simulink model "UZ_EnDat_be4_diffrework"  (R2023b)
settings: Solver=FixedStepDiscrete  StartTime=0  StopTime=0.002  RelTol=1e-3
model workspace (MAT data in the model file):
  Select = 0
libraries: hdlsllib x207, simulink x17, simulink_extras x3
(part 2 of 5)

== system UZ_EnDat_be4_diffrework/UZ_ENDAT/CLKCNTER_NOSTOP ==
  CLK : Inport
  CLK2CNT : Inport  Port=2
  ResetCNT : Inport  Port=3  OutDataTypeStr=boolean
  Delay1 : Delay  DelayLength=1
  Positional_Counter : Subsystem  TreatAsAtomicUnit=on
      settings: LibrarySourceBlock=|
      | hdlsllib/Ports &
      | Subsystems/Triggered
      | Subsystem
  SetZero32modified : Subsystem
  CNT : Outport
  wires:
  Delay1/1 -> SetZero32modified/1(valin), CNT/1
  CLK2CNT/1 -> Positional_Counter/Trigger
  ResetCNT/1 -> SetZero32modified/2(setzero)
  Positional_Counter/1(divider) -> Delay1/1
  CLK/1 -> SetZero32modified/Trigger
  SetZero32modified/1(valueout) -> Positional_Counter/1(valueout)

== system UZ_EnDat_be4_diffrework/UZ_ENDAT/CLKCNTER_RAMPUP ==
  CLK : Inport
  CLK2CNT : Inport  Port=2
  ResetCNT : Inport  Port=3  OutDataTypeStr=boolean
  Delay1 : Delay  DelayLength=1
  Positional_Counter : Subsystem  TreatAsAtomicUnit=on
      settings: LibrarySourceBlock=|
      | hdlsllib/Ports &
      | Subsystems/Triggered
      | Subsystem
  SetZero32modified : Subsystem
  CNT : Outport
  wires:
  CLK2CNT/1 -> Positional_Counter/Trigger
  Delay1/1 -> Positional_Counter/1(valueout), CNT/1
  SetZero32modified/1(valueout) -> Delay1/1
  CLK/1 -> SetZero32modified/Trigger
  Positional_Counter/1(divider) -> SetZero32modified/1(valin)
  ResetCNT/1 -> SetZero32modified/2(setzero)

== system UZ_EnDat_be4_diffrework/UZ_ENDAT/CLKDIV1 ==
  CLK1 : Inport  OutDataTypeStr=boolean
  Delay : Delay  DelayLength=1
  Logical Operator1 : Logic  Operator=NOT  AllPortsSameDT=off  OutDataTypeStr=boolean
  Triggered Subsystem : Subsystem  TreatAsAtomicUnit=on
      settings: LibrarySourceBlock=|
      | hdlsllib/Ports &
      | Subsystems/Triggered
      | Subsystem
  CLK/2 : Outport  OutDataTypeStr=boolean  VectorParamsAs1DForOutWhenUnconnected=off
  wires:
  Logical Operator1/1 -> CLK/2/1, Delay/1
  CLK1/1 -> Triggered Subsystem/Trigger
  Triggered Subsystem/1(OUT) -> Logical Operator1/1
  Delay/1 -> Triggered Subsystem/1(IN)

== system UZ_EnDat_be4_diffrework/UZ_ENDAT/CLKDIV2 ==
  CLK1 : Inport  OutDataTypeStr=boolean
  Delay : Delay  DelayLength=1
  Logical Operator1 : Logic  Operator=NOT  AllPortsSameDT=off  OutDataTypeStr=boolean
  Triggered Subsystem : Subsystem  TreatAsAtomicUnit=on
      settings: LibrarySourceBlock=|
      | hdlsllib/Ports &
      | Subsystems/Triggered
      | Subsystem
  CLK/2 : Outport  OutDataTypeStr=boolean  VectorParamsAs1DForOutWhenUnconnected=off
  wires:
  Logical Operator1/1 -> CLK/2/1, Delay/1
  CLK1/1 -> Triggered Subsystem/Trigger
  Triggered Subsystem/1(OUT) -> Logical Operator1/1
  Delay/1 -> Triggered Subsystem/1(IN)

== system UZ_EnDat_be4_diffrework/UZ_ENDAT/CLKDIV3 ==
  CLK1 : Inport  OutDataTypeStr=boolean
  Delay : Delay  DelayLength=1
  Logical Operator1 : Logic  Operator=NOT  AllPortsSameDT=off  OutDataTypeStr=boolean
  Triggered Subsystem : Subsystem  TreatAsAtomicUnit=on
      settings: LibrarySourceBlock=|
      | hdlsllib/Ports &
      | Subsystems/Triggered
      | Subsystem
  CLK/2 : Outport  OutDataTypeStr=boolean  VectorParamsAs1DForOutWhenUnconnected=off
  wires:
  Logical Operator1/1 -> CLK/2/1, Delay/1
  CLK1/1 -> Triggered Subsystem/Trigger
  Triggered Subsystem/1(OUT) -> Logical Operator1/1
  Delay/1 -> Triggered Subsystem/1(IN)

== system UZ_EnDat_be4_diffrework/UZ_ENDAT/CLKDIV4 ==
  CLK1 : Inport  OutDataTypeStr=boolean
  Delay : Delay  DelayLength=1
  Logical Operator1 : Logic  Operator=NOT  AllPortsSameDT=off  OutDataTypeStr=boolean
  Triggered Subsystem : Subsystem  TreatAsAtomicUnit=on
      settings: LibrarySourceBlock=|
      | hdlsllib/Ports &
      | Subsystems/Triggered
      | Subsystem
  CLK/2 : Outport  OutDataTypeStr=boolean  VectorParamsAs1DForOutWhenUnconnected=off
  wires:
  Logical Operator1/1 -> CLK/2/1, Delay/1
  CLK1/1 -> Triggered Subsystem/Trigger
  Triggered Subsystem/1(OUT) -> Logical Operator1/1
  Delay/1 -> Triggered Subsystem/1(IN)

== system UZ_EnDat_be4_diffrework/UZ_ENDAT/CLKDIV5 ==
  CLK1 : Inport  OutDataTypeStr=boolean
  Delay : Delay  DelayLength=1
  Logical Operator1 : Logic  Operator=NOT  AllPortsSameDT=off  OutDataTypeStr=boolean
  Triggered Subsystem : Subsystem  TreatAsAtomicUnit=on
      settings: LibrarySourceBlock=|
      | hdlsllib/Ports &
      | Subsystems/Triggered
      | Subsystem
  CLK/2 : Outport  OutDataTypeStr=boolean  VectorParamsAs1DForOutWhenUnconnected=off
  wires:
  Logical Operator1/1 -> CLK/2/1, Delay/1
  CLK1/1 -> Triggered Subsystem/Trigger
  Triggered Subsystem/1(OUT) -> Logical Operator1/1
  Delay/1 -> Triggered Subsystem/1(IN)

== system UZ_EnDat_be4_diffrework/UZ_ENDAT/CLKDIV6 ==
  CLK1 : Inport  OutDataTypeStr=boolean
  Delay : Delay  DelayLength=1
  Logical Operator1 : Logic  Operator=NOT  AllPortsSameDT=off  OutDataTypeStr=boolean
  Triggered Subsystem : Subsystem  TreatAsAtomicUnit=on
      settings: LibrarySourceBlock=|
      | hdlsllib/Ports &
      | Subsystems/Triggered
      | Subsystem
  CLK/2 : Outport  OutDataTypeStr=boolean  VectorParamsAs1DForOutWhenUnconnected=off
  wires:
  Logical Operator1/1 -> CLK/2/1, Delay/1
  CLK1/1 -> Triggered Subsystem/Trigger
  Triggered Subsystem/1(OUT) -> Logical Operator1/1
  Delay/1 -> Triggered Subsystem/1(IN)

== system UZ_EnDat_be4_diffrework/UZ_ENDAT/CLKDIV7 ==
  CLK1 : Inport  OutDataTypeStr=boolean
  Delay : Delay  DelayLength=1
  Logical Operator1 : Logic  Operator=NOT  AllPortsSameDT=off  OutDataTypeStr=boolean
  Triggered Subsystem : Subsystem  TreatAsAtomicUnit=on
      settings: LibrarySourceBlock=|
      | hdlsllib/Ports &
      | Subsystems/Triggered
      | Subsystem
  CLK/2 : Outport  OutDataTypeStr=boolean  VectorParamsAs1DForOutWhenUnconnected=off
  wires:
  Logical Operator1/1 -> CLK/2/1, Delay/1
  CLK1/1 -> Triggered Subsystem/Trigger
  Triggered Subsystem/1(OUT) -> Logical Operator1/1
  Delay/1 -> Triggered Subsystem/1(IN)

== system UZ_EnDat_be4_diffrework/UZ_ENDAT/CLKDIV8 ==
  CLK1 : Inport  OutDataTypeStr=boolean
  Delay : Delay  DelayLength=1
  Logical Operator1 : Logic  Operator=NOT  AllPortsSameDT=off  OutDataTypeStr=boolean
  Triggered Subsystem : Subsystem  TreatAsAtomicUnit=on
      settings: LibrarySourceBlock=|
      | hdlsllib/Ports &
      | Subsystems/Triggered
      | Subsystem
  CLK/2 : Outport  OutDataTypeStr=boolean  VectorParamsAs1DForOutWhenUnconnected=off
  wires:
  Logical Operator1/1 -> CLK/2/1, Delay/1
  CLK1/1 -> Triggered Subsystem/Trigger
  Triggered Subsystem/1(OUT) -> Logical Operator1/1
  Delay/1 -> Triggered Subsystem/1(IN)

== system UZ_EnDat_be4_diffrework/UZ_ENDAT/CLKDIV9 ==
  CLK1 : Inport  OutDataTypeStr=boolean
  Delay : Delay  DelayLength=1
  Logical Operator1 : Logic  Operator=NOT  AllPortsSameDT=off  OutDataTypeStr=boolean
  Triggered Subsystem : Subsystem  TreatAsAtomicUnit=on
      settings: LibrarySourceBlock=|
      | hdlsllib/Ports &
      | Subsystems/Triggered
      | Subsystem
  CLK/2 : Outport  OutDataTypeStr=boolean  VectorParamsAs1DForOutWhenUnconnected=off
  wires:
  Logical Operator1/1 -> CLK/2/1, Delay/1
  CLK1/1 -> Triggered Subsystem/Trigger
  Triggered Subsystem/1(OUT) -> Logical Operator1/1
  Delay/1 -> Triggered Subsystem/1(IN)

== system UZ_EnDat_be4_diffrework/UZ_ENDAT/CONTROLWORDRAW ==
  CLK : Inport
  DATA : Inport  Port=2
  WORDTOBOOL : Subsystem  TreatAsAtomicUnit=on
  DATAOUT0 : Outport  VectorParamsAs1DForOutWhenUnconnected=off
  DATAOUT1 : Outport  Port=2  VectorParamsAs1DForOutWhenUnconnected=off
  DATAOUT2 : Outport  Port=3  VectorParamsAs1DForOutWhenUnconnected=off
  DATAOUT3 : Outport  Port=4  VectorParamsAs1DForOutWhenUnconnected=off
  DATAOUT4 : Outport  Port=5  VectorParamsAs1DForOutWhenUnconnected=off
  DATAOUT5 : Outport  Port=6  VectorParamsAs1DForOutWhenUnconnected=off
  DATAOUT6 : Outport  Port=7  VectorParamsAs1DForOutWhenUnconnected=off
  DATAOUT7 : Outport  Port=8  VectorParamsAs1DForOutWhenUnconnected=off
  DATAOUT8 : Outport  Port=9  VectorParamsAs1DForOutWhenUnconnected=off
  DATAOUT9 : Outport  Port=10  VectorParamsAs1DForOutWhenUnconnected=off
  DATAOUT10 : Outport  Port=11  VectorParamsAs1DForOutWhenUnconnected=off
  DATAOUT11 : Outport  Port=12  VectorParamsAs1DForOutWhenUnconnected=off
  DATAOUT12 : Outport  Port=13  VectorParamsAs1DForOutWhenUnconnected=off
  DATAOUT13 : Outport  Port=14  VectorParamsAs1DForOutWhenUnconnected=off
  DATAOUT14 : Outport  Port=15  VectorParamsAs1DForOutWhenUnconnected=off
  DATAOUT15 : Outport  Port=16  VectorParamsAs1DForOutWhenUnconnected=off
  wires:
  DATA/1 -> WORDTOBOOL/1(DATAIN)
  CLK/1 -> WORDTOBOOL/Trigger
  WORDTOBOOL/1(DATAOUT0) -> DATAOUT0/1
  WORDTOBOOL/2(DATAOUT1) -> DATAOUT1/1
  WORDTOBOOL/3(DATAOUT2) -> DATAOUT2/1
  WORDTOBOOL/4(DATAOUT3) -> DATAOUT3/1
  WORDTOBOOL/6(DATAOUT5) -> DATAOUT5/1
  WORDTOBOOL/5(DATAOUT4) -> DATAOUT4/1
  WORDTOBOOL/7(DATAOUT6) -> DATAOUT6/1
  WORDTOBOOL/8(DATAOUT7) -> DATAOUT7/1
  WORDTOBOOL/10(DATAOUT9) -> DATAOUT9/1
  WORDTOBOOL/9(DATAOUT8) -> DATAOUT8/1
  WORDTOBOOL/11(DATAOUT10) -> DATAOUT10/1
  WORDTOBOOL/12(DATAOUT11) -> DATAOUT11/1
  WORDTOBOOL/14(DATAOUT13) -> DATAOUT13/1
  WORDTOBOOL/13(DATAOUT12) -> DATAOUT12/1
  WORDTOBOOL/15(DATAOUT14) -> DATAOUT14/1
  WORDTOBOOL/16(DATAOUT15) -> DATAOUT15/1

== system UZ_EnDat_be4_diffrework/UZ_ENDAT/CONTROLWORDSTORED ==
  CLK : Inport
  DATA : Inport  Port=2
  WORDTOBOOL : Subsystem  TreatAsAtomicUnit=on
  DATAOUT0 : Outport  VectorParamsAs1DForOutWhenUnconnected=off
  DATAOUT1 : Outport  Port=2  VectorParamsAs1DForOutWhenUnconnected=off
  DATAOUT2 : Outport  Port=3  VectorParamsAs1DForOutWhenUnconnected=off
  DATAOUT3 : Outport  Port=4  VectorParamsAs1DForOutWhenUnconnected=off
  DATAOUT4 : Outport  Port=5  VectorParamsAs1DForOutWhenUnconnected=off
  DATAOUT5 : Outport  Port=6  VectorParamsAs1DForOutWhenUnconnected=off
  DATAOUT6 : Outport  Port=7  VectorParamsAs1DForOutWhenUnconnected=off
  DATAOUT7 : Outport  Port=8  VectorParamsAs1DForOutWhenUnconnected=off
  DATAOUT8 : Outport  Port=9  VectorParamsAs1DForOutWhenUnconnected=off
  DATAOUT9 : Outport  Port=10  VectorParamsAs1DForOutWhenUnconnected=off
  DATAOUT10 : Outport  Port=11  VectorParamsAs1DForOutWhenUnconnected=off
  DATAOUT11 : Outport  Port=12  VectorParamsAs1DForOutWhenUnconnected=off
  DATAOUT12 : Outport  Port=13  VectorParamsAs1DForOutWhenUnconnected=off
  DATAOUT13 : Outport  Port=14  VectorParamsAs1DForOutWhenUnconnected=off
  DATAOUT14 : Outport  Port=15  VectorParamsAs1DForOutWhenUnconnected=off
  DATAOUT15 : Outport  Port=16  VectorParamsAs1DForOutWhenUnconnected=off
  wires:
  DATA/1 -> WORDTOBOOL/1(DATAIN)
  CLK/1 -> WORDTOBOOL/Trigger
  WORDTOBOOL/1(DATAOUT0) -> DATAOUT0/1
  WORDTOBOOL/2(DATAOUT1) -> DATAOUT1/1
  WORDTOBOOL/3(DATAOUT2) -> DATAOUT2/1
  WORDTOBOOL/4(DATAOUT3) -> DATAOUT3/1
  WORDTOBOOL/6(DATAOUT5) -> DATAOUT5/1
  WORDTOBOOL/5(DATAOUT4) -> DATAOUT4/1
  WORDTOBOOL/7(DATAOUT6) -> DATAOUT6/1
  WORDTOBOOL/8(DATAOUT7) -> DATAOUT7/1
  WORDTOBOOL/10(DATAOUT9) -> DATAOUT9/1
  WORDTOBOOL/9(DATAOUT8) -> DATAOUT8/1
  WORDTOBOOL/11(DATAOUT10) -> DATAOUT10/1
  WORDTOBOOL/12(DATAOUT11) -> DATAOUT11/1
  WORDTOBOOL/14(DATAOUT13) -> DATAOUT13/1
  WORDTOBOOL/13(DATAOUT12) -> DATAOUT12/1
  WORDTOBOOL/15(DATAOUT14) -> DATAOUT14/1
  WORDTOBOOL/16(DATAOUT15) -> DATAOUT15/1

== system UZ_EnDat_be4_diffrework/UZ_ENDAT/CRC_Check ==
  set : Inport
  data : Inport  Port=2  OutDataTypeStr=boolean
  clk : Inport  Port=3  OutDataTypeStr=boolean
  Constant : Constant  OutDataTypeStr=boolean  SampleTime=-1
  Constant1 : Constant  Value=0  OutDataTypeStr=boolean  SampleTime=-1
  DFF1 : Subsystem
  DFF2 : Subsystem
  DFF3 : Subsystem
  DFF4 : Subsystem
  DFF5 : Subsystem
  DFF6 : Subsystem  Commented=on
  FF0 : Subsystem  Commented=on  TreatAsAtomicUnit=on
      settings: LibrarySourceBlock=|
      | hdlsllib/Ports &
      | Subsystems/Triggered
      | Subsystem
  Logical Operator : Logic  Operator=OR  AllPortsSameDT=off  OutDataTypeStr=boolean
  Logical Operator{1..2,5..6} (4 alike) : Logic  AllPortsSameDT=off  OutDataTypeStr=boolean
  Logical Operator3 : Logic  Operator=NOT  AllPortsSameDT=off  OutDataTypeStr=boolean
  Logical Operator4 : Logic  Operator=NOT  AllPortsSameDT=off  OutDataTypeStr=boolean
  Memory : Memory  InheritSampleTime=on
  Memory1 : Memory  InheritSampleTime=on
  Relational Operator : RelationalOperator  Operator===  OutDataTypeStr=boolean  InputSameDT=off
  Relational Operator1 : RelationalOperator  Operator===  OutDataTypeStr=boolean  InputSameDT=off
  Relational Operator2 : RelationalOperator  Operator===  OutDataTypeStr=boolean  InputSameDT=off
  Terminator{,1..3} (4 alike) : Terminator
  crc : Outport
  CRC1 : Outport  Port=2
  CRC2 : Outport  Port=3
  CRC3 : Outport  Port=4
  CRC4 : Outport  Port=5
  CRC5 : Outport  Port=6
  wires:
  Logical Operator/1 -> crc/1
  Logical Operator2/1 -> Logical Operator/2
  Logical Operator1/1 -> Logical Operator/1
  data/1 -> Relational Operator/2, Logical Operator1/1
  Logical Operator3/1 -> Logical Operator1/2
  Logical Operator4/1 -> Logical Operator3/1, Logical Operator2/2
  Logical Operator5/1 -> Memory1/1
  Relational Operator/1 -> DFF1/3(D), Logical Operator6/1
  clk/1 -> DFF1/2(CLK), DFF2/2(CLK), DFF3/2(CLK), DFF5/2(CLK), DFF4/2(CLK)
  set/1 -> Logical Operator6/2, Logical Operator5/2, Logical Operator4/1
  DFF1/1(OQ) -> Relational Operator1/1, CRC1/1
  Logical Operator6/1 -> Memory/1
  Relational Operator1/1 -> DFF2/3(D)
  Relational Operator2/1 -> DFF4/3(D)
  DFF3/1(OQ) -> CRC3/1, Relational Operator2/1
  DFF4/1(OQ) -> DFF5/3(D), CRC4/1
  DFF5/2(NOQ) -> Logical Operator2/1
  DFF5/1(OQ) -> Logical Operator5/1, CRC5/1
  DFF2/1(OQ) -> DFF3/3(D), CRC2/1
  DFF1/2(NOQ) -> Terminator/1
  DFF2/2(NOQ) -> Terminator1/1
  DFF3/2(NOQ) -> Terminator2/1
  DFF4/2(NOQ) -> Terminator3/1
  Constant/1 -> DFF3/1(SET), DFF5/1(SET), DFF4/1(SET), DFF2/1(SET), DFF1/1(SET)
  Constant1/1 -> DFF5/4(RST), DFF4/4(RST), DFF3/4(RST), DFF2/4(RST), DFF1/4(RST)
  Memory/1 -> Relational Operator2/2, Relational Operator1/2
  Memory1/1 -> Relational Operator/1

== system UZ_EnDat_be4_diffrework/UZ_ENDAT/DATA2CLOCKSYNCER ==
  In1 : Inport
  FAKTOR : Inport  Port=2
  Constant : Constant  Value=100  OutDataTypeStr=uint16  SampleTime=-1
  Constant1 : Constant  Value=45  OutDataTypeStr=uint16  SampleTime=-1
  Constant2 : Constant  Value=2  OutDataTypeStr=uint16  SampleTime=-1
  Constant23 : Constant  Value=20  OutDataTypeStr=uint16  SampleTime=-1
  Constant24 : Constant  Value=29  OutDataTypeStr=uint16  SampleTime=-1
  Constant3 : Constant  Value=12  OutDataTypeStr=uint16  SampleTime=-1
  Constant4 : Constant  Value=4  OutDataTypeStr=uint16  SampleTime=-1
  Constant7 : Constant  Value=8  OutDataTypeStr=uint16  SampleTime=-1
  Display15 : Display
  Divide : Product  Inputs=*/  OutDataTypeStr=uint16  RndMeth=Simplest  SaturateOnIntegerOverflow=on  LockScale=on
  Multiport Switch1 : MultiPortSwitch  DataPortOrder=Zero-based contiguous  Inputs=7  DataPortIndices={8,16,32,64}  zeroidx=on  SaturateOnIntegerOverflow=off  InputSameDT=off
  Product : Product  RndMeth=Simplest  SaturateOnIntegerOverflow=on  OutDataTypeStr=Inherit: Same as first input
  Out1 : Outport
  wires:
  In1/1 -> Multiport Switch1/1
  FAKTOR/1 -> Product/2
  Constant/1 -> Divide/2
  Multiport Switch1/1 -> Product/1
  Product/1 -> Divide/1
  Constant2/1 -> Multiport Switch1/2
  Constant4/1 -> Multiport Switch1/3
  Constant7/1 -> Multiport Switch1/4
  Constant3/1 -> Multiport Switch1/5
  Constant23/1 -> Multiport Switch1/6
  Constant24/1 -> Multiport Switch1/7
  Constant1/1 -> Multiport Switch1/8
  Divide/1 -> Display15/1, Out1/1

== system UZ_EnDat_be4_diffrework/UZ_ENDAT/DATA2CLOCKSYNCER1 ==
  In1 : Inport
  FAKTOR : Inport  Port=2
  Constant : Constant  Value=9999  OutDataTypeStr=uint16  SampleTime=-1
  Constant1 : Constant  Value=384  OutDataTypeStr=uint16  SampleTime=-1
  Constant2 : Constant  Value=5  OutDataTypeStr=uint16  SampleTime=-1
  Constant23 : Constant  Value=96  OutDataTypeStr=uint16  SampleTime=-1
  Constant24 : Constant  Value=192  OutDataTypeStr=uint16  SampleTime=-1
  Constant3 : Constant  Value=48  OutDataTypeStr=uint16  SampleTime=-1
  Constant4 : Constant  Value=11  OutDataTypeStr=uint16  SampleTime=-1
  Constant7 : Constant  Value=23  OutDataTypeStr=uint16  SampleTime=-1
  Display15 : Display
  Divide : Product  Inputs=*/  OutDataTypeStr=uint16  RndMeth=Simplest  SaturateOnIntegerOverflow=on  LockScale=on
  Multiport Switch1 : MultiPortSwitch  DataPortOrder=Zero-based contiguous  Inputs=7  DataPortIndices={8,16,32,64}  zeroidx=on  SaturateOnIntegerOverflow=off  InputSameDT=off
  Product : Product  RndMeth=Simplest  SaturateOnIntegerOverflow=on  OutDataTypeStr=Inherit: Same as first input
  Out1 : Outport
  wires:
  In1/1 -> Multiport Switch1/1
  FAKTOR/1 -> Product/2
  Constant/1 -> Divide/2
  Multiport Switch1/1 -> Product/1
  Product/1 -> Divide/1
  Constant2/1 -> Multiport Switch1/2
  Constant4/1 -> Multiport Switch1/3
  Constant7/1 -> Multiport Switch1/4
  Constant3/1 -> Multiport Switch1/5
  Constant23/1 -> Multiport Switch1/6
  Constant24/1 -> Multiport Switch1/7
  Constant1/1 -> Multiport Switch1/8
  Divide/1 -> Display15/1, Out1/1

== system UZ_EnDat_be4_diffrework/UZ_ENDAT/DATAFLOWCHGER ==
  CLKSEL : Inport
  FACTOR : Inport  Port=2
  Constant : Constant  Value=100  OutDataTypeStr=uint16  SampleTime=-1
  Constant{14..18,27..28} (7 alike) : Constant  Value=10  OutDataTypeStr=uint16  SampleTime=-1
  Divide : Product  Inputs=*/  InputSameDT=on  OutDataTypeStr=uint16  RndMeth=Simplest  SaturateOnIntegerOverflow=on
  Multiport Switch2 : MultiPortSwitch  DataPortOrder=Zero-based contiguous  Inputs=7  DataPortIndices={8,16,32,64}  zeroidx=on  SaturateOnIntegerOverflow=off  InputSameDT=off
  Product : Product  RndMeth=Simplest  SaturateOnIntegerOverflow=on  OutDataTypeStr=Inherit: Same as first input
  Output : Outport
  wires:
  Product/1 -> Divide/1
  CLKSEL/1 -> Multiport Switch2/1
  FACTOR/1 -> Product/2
  Constant/1 -> Divide/2
  Divide/1 -> Output/1
  Multiport Switch2/1 -> Product/1
  Constant15/1 -> Multiport Switch2/2
  Constant16/1 -> Multiport Switch2/3
  Constant17/1 -> Multiport Switch2/4
  Constant18/1 -> Multiport Switch2/5
  Constant27/1 -> Multiport Switch2/6
  Constant28/1 -> Multiport Switch2/7
  Constant14/1 -> Multiport Switch2/8

== system UZ_EnDat_be4_diffrework/UZ_ENDAT/INITIALOFF ==
  CLKAUX : Inport
  CLK : Inport  Port=2
  DATAWR : Inport  Port=3
  DATA : Inport  Port=4
  CLKWR : Inport  Port=5
  FACTOR : Inport  Port=6
  CLKCNTER_FAST : Subsystem
      settings: LibrarySourceBlock=|
      | hdlsllib/Ports &
      | Subsystems/Subsystem
  Constant : Constant  Value=0  OutDataTypeStr=boolean  SampleTime=-1
  Multiport Switch{,1..3} (4 alike) : MultiPortSwitch  DataPortOrder=Zero-based contiguous  Inputs=2  zeroidx=on  SaturateOnIntegerOverflow=off  InputSameDT=off
  Relational Operator : RelationalOperator  Operator=<  OutDataTypeStr=boolean  InputSameDT=off
  Subsystem6 : Subsystem
  CLK_OUT : Outport
  DATAWR_OUT : Outport  Port=2
  DATA_OUT : Outport  Port=3
  CLKWR_OUT : Outport  Port=4
  wires:
  CLKCNTER_FAST/1(CNT) -> Relational Operator/1
  Relational Operator/1 -> Multiport Switch3/1, Multiport Switch2/1, Multiport Switch1/1, Multiport Switch/1
  CLK/1 -> Multiport Switch/2
  Multiport Switch/1 -> CLK_OUT/1
  CLKAUX/1 -> CLKCNTER_FAST/1(CLK)
  Constant/1 -> Multiport Switch3/3, Multiport Switch2/3, Multiport Switch1/3, Multiport Switch/3
  Multiport Switch1/1 -> DATAWR_OUT/1
  Multiport Switch2/1 -> DATA_OUT/1
  Multiport Switch3/1 -> CLKWR_OUT/1
  DATAWR/1 -> Multiport Switch1/2
  DATA/1 -> Multiport Switch2/2
  CLKWR/1 -> Multiport Switch3/2
  Subsystem6/1(out) -> Relational Operator/2
  FACTOR/1 -> Subsystem6/1(FACTOR)

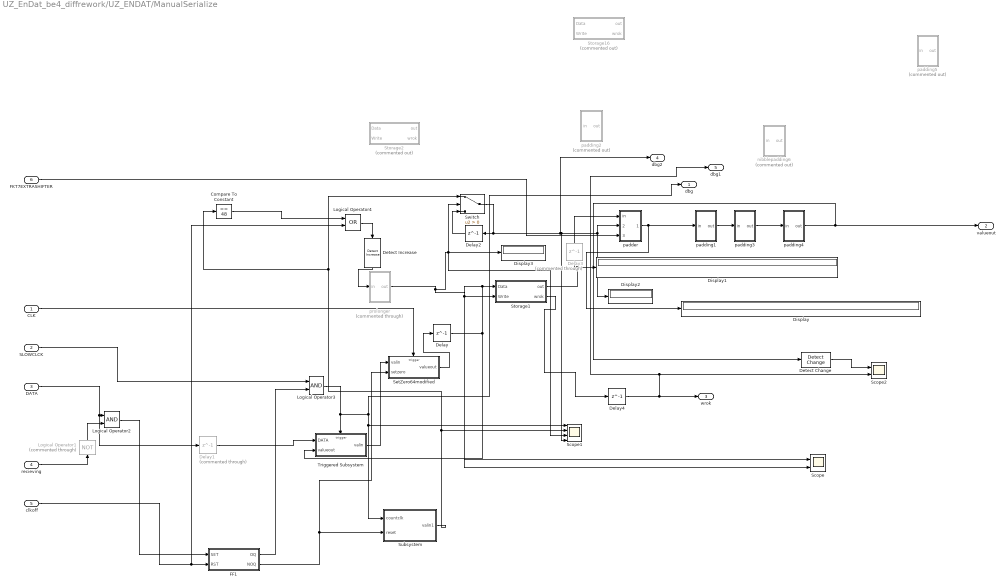
== system UZ_EnDat_be4_diffrework/UZ_ENDAT/ManualSerialize ==
  CLK : Inport
  SLOWCLCK : Inport  Port=2
  DATA : Inport  Port=3
  recieving : Inport  Port=4  OutMin=0  OutMax=1  OutDataTypeStr=boolean
  clkoff : Inport  Port=5  OutMin=0  OutMax=1  OutDataTypeStr=boolean
  FKT7EXTRASHIFTER : Inport  Port=6
  Compare To Constant : hdlsllib/Logic and Bit Operations/Compare To Constant  relop===  const=48  OutDataTypeStr=boolean
  Delay : Delay  DelayLength=1
  Delay1 : Delay  Commented=through  DelayLength=1
  Delay2 : Delay  DelayLength=1
  Delay3 : Delay  Commented=through  DelayLength=1
  Delay4 : Delay  DelayLength=1
  Detect Change : simulink/Logic and Bit Operations/Detect Change  vinit=0  OutDataTypeStr=boolean
  Detect Increase : simulink/Logic and Bit Operations/Detect Increase  vinit=0.0  OutDataTypeStr=boolean
      settings: LibrarySourceBlock=|
      | hdlsllib/Logic and Bit
      | Operations/Detect
      | Increase
  Display{,1..3} (4 alike) : Display
      Display settings: Format=binary (Stored Integer)
      Display1 settings: Format=binary (Stored Integer)
  FF1 : Subsystem  TreatAsAtomicUnit=on
      settings: LibrarySourceBlock=|
      | hdlsllib/Ports &
      | Subsystems/Triggered
      | Subsystem
  Logical Operator1 : Logic  Commented=through  Operator=NOT  AllPortsSameDT=off  OutDataTypeStr=boolean
  Logical Operator2 : Logic  AllPortsSameDT=off  OutDataTypeStr=boolean
  Logical Operator3 : Logic  AllPortsSameDT=off  OutDataTypeStr=boolean
  Logical Operator4 : Logic  Operator=OR  AllPortsSameDT=off  OutDataTypeStr=boolean
  Scope : Scope  NumInputPorts=2
  Scope1 : Scope  NumInputPorts=4
  Scope2 : Scope  NumInputPorts=2
  SetZero64modified : Subsystem
  Storage1 : Subsystem
      settings: LibrarySourceBlock=|
      | hdlsllib/Ports &
      | Subsystems/Subsystem
  Storage16 : Subsystem  Commented=on
      settings: LibrarySourceBlock=|
      | hdlsllib/Ports &
      | Subsystems/Subsystem
  Storage2 : Subsystem  Commented=on
      settings: LibrarySourceBlock=|
      | hdlsllib/Ports &
      | Subsystems/Subsystem
  Subsystem : Subsystem
  Switch : Switch  Criteria=u2 > Threshold  SaturateOnIntegerOverflow=off  InputSameDT=off
  Triggered Subsystem : Subsystem  TreatAsAtomicUnit=on
      settings: LibrarySourceBlock=|
      | hdlsllib/Ports &
      | Subsystems/Triggered
      | Subsystem
  nibblepadding6 : Subsystem  Commented=on
  padder : Subsystem
  padding1 : Subsystem
  padding2 : Subsystem  Commented=on
  padding3 : Subsystem
  padding4 : Subsystem
  padding5 : Subsystem  Commented=on
  prolonger : Subsystem  Commented=through
  dbg : Outport  OutDataTypeStr=boolean  VectorParamsAs1DForOutWhenUnconnected=off
  valueout : Outport  Port=2  OutDataTypeStr=uint64
  wrok : Outport  Port=3  OutDataTypeStr=boolean
  dbg2 : Outport  Port=4  OutDataTypeStr=uint8  VectorParamsAs1DForOutWhenUnconnected=off
  dbg1 : Outport  Port=5  OutDataTypeStr=boolean  VectorParamsAs1DForOutWhenUnconnected=off
  wires:
  SetZero64modified/1(valueout) -> Delay/1
  CLK/1 -> SetZero64modified/Trigger
  SLOWCLCK/1 -> Logical Operator3/1
  Triggered Subsystem/1(valin) -> SetZero64modified/1(valin)
  Storage1/2(wrok) -> Delay4/1
  Logical Operator3/1 -> dbg/1, Subsystem/1(countclk), Scope1/1, Triggered Subsystem/Trigger
  Logical Operator2/1 -> FF1/1(SET)
  FF1/1(OQ) -> Logical Operator3/2
  Logical Operator1/1 -> Logical Operator2/2
  recieving/1 -> Logical Operator1/1
  FF1/2(NOQ) -> Subsystem/2(reset), SetZero64modified/2(setzero)
  DATA/1 -> Delay1/1, Logical Operator2/1
  Compare To Constant/1 -> Logical Operator4/1
  Delay2/1 -> Switch/3
  clkoff/1 -> Logical Operator4/2, FF1/2(RST)
  Logical Operator4/1 -> Detect Increase/1
  Subsystem/1(valin1) -> Scope1/2, Switch/1, Compare To Constant/1
  Delay1/1 -> Triggered Subsystem/1(DATA)
  Delay/1 -> Storage1/1(Data), Scope/2, Triggered Subsystem/2(valueout)
  padding1/1(out) -> padding3/1(in)
  padder/1(out) -> padding1/1(in), Display/1
  Storage1/1(out) -> Delay3/1, Display1/1
  padding3/1(out) -> padding4/1(in)
  Delay3/1 -> padder/1(in)
  prolonger/1(out) -> Storage1/2(Write), Scope/1, Switch/2, Scope1/3, Display3/1
  Detect Increase/1 -> prolonger/1(in)
  padding4/1(out) -> Detect Change/1, valueout/1
  Switch/1 -> Delay2/1, Scope1/4, padder/2(CTR), Display2/1, dbg2/1
  Detect Change/1 -> Scope2/1
  Delay4/1 -> dbg1/1, Scope2/2, wrok/1
  FKT7EXTRASHIFTER/1 -> padder/3(in1)

== system UZ_EnDat_be4_diffrework/UZ_ENDAT/OUTPUTCONTROLCONTINIOUS ==
  CLKCNT : Inport
  CLKS2DATAFLOWCHG : Inport  Port=2
  CLK2ENDOFTRANSMISSION : Inport  Port=3
  OPENCOM : Inport  Port=4
  CLKCNTNOSTOP : Inport  Port=5
  RECOVERYTIME : Inport  Port=6  OutDataTypeStr=uint16
  Add : Sum  OutDataTypeStr=uint16  AccumDataTypeStr=uint16
  Constant : Constant  Value=0  OutDataTypeStr=uint8  SampleTime=-1
  Logical Operator : Logic  Operator=OR  AllPortsSameDT=off  OutDataTypeStr=boolean
  Logical Operator1 : Logic  AllPortsSameDT=off  OutDataTypeStr=boolean
  Logical Operator6 : Logic  Operator=NOT  Inputs=3  AllPortsSameDT=off  OutDataTypeStr=boolean
  Relational Operator : RelationalOperator  Operator=<=  OutDataTypeStr=boolean  InputSameDT=off
  Relational Operator1 : RelationalOperator  OutDataTypeStr=boolean  InputSameDT=off
  Relational Operator2 : RelationalOperator  OutDataTypeStr=boolean  InputSameDT=off
  Relational Operator3 : RelationalOperator  OutDataTypeStr=boolean  InputSameDT=off
  CLKOFF : Outport  OutDataTypeStr=boolean
  DATAINV : Outport  Port=2  OutDataTypeStr=boolean
  RESETCNT : Outport  Port=3  OutDataTypeStr=boolean
  wires:
  CLKCNT/1 -> Relational Operator1/1, Relational Operator2/1, Relational Operator/1
  CLKS2DATAFLOWCHG/1 -> Relational Operator/2
  Relational Operator/1 -> Logical Operator1/1
  CLK2ENDOFTRANSMISSION/1 -> Add/1, Relational Operator1/2
  Relational Operator1/1 -> Logical Operator/2
  Logical Operator/1 -> CLKOFF/1
  OPENCOM/1 -> Logical Operator6/1
  Logical Operator6/1 -> Logical Operator/1
  Relational Operator2/1 -> Logical Operator1/2
  Constant/1 -> Relational Operator2/2
  Logical Operator1/1 -> DATAINV/1
  RECOVERYTIME/1 -> Add/2
  Add/1 -> Relational Operator3/2
  Relational Operator3/1 -> RESETCNT/1
  CLKCNTNOSTOP/1 -> Relational Operator3/1

== system UZ_EnDat_be4_diffrework/UZ_ENDAT/RECOVERYTIMESELECTOR ==
  note: 200khz = 6
      | 1,5mhz = 12
      | 3 mhz = 8
  In1 : Inport
  FAKTOR : Inport  Port=2
  Constant : Constant  Value=100  OutDataTypeStr=uint16  SampleTime=-1
  Constant19 : Constant  Value=96  OutDataTypeStr=uint16  SampleTime=-1
  Constant20 : Constant  Value=48  OutDataTypeStr=uint16  SampleTime=-1
  Constant21 : Constant  Value=192  OutDataTypeStr=uint16  SampleTime=-1
  Constant22 : Constant  Value=255  OutDataTypeStr=uint16  SampleTime=-1
  Constant25 : Constant  Value=24  OutDataTypeStr=uint16  SampleTime=-1
  Constant26 : Constant  Value=12  OutDataTypeStr=uint16  SampleTime=-1
  Constant5 : Constant  Value=6  OutDataTypeStr=uint16  SampleTime=-1
  Divide : Product  Inputs=*/  InputSameDT=on  OutDataTypeStr=uint16  RndMeth=Simplest  SaturateOnIntegerOverflow=on
  Multiport Switch3 : MultiPortSwitch  DataPortOrder=Zero-based contiguous  Inputs=7  DataPortIndices={8,16,32,64}  zeroidx=on  SaturateOnIntegerOverflow=off  InputSameDT=off
  Product : Product  RndMeth=Simplest  SaturateOnIntegerOverflow=on  OutDataTypeStr=Inherit: Same as first input
  Out1 : Outport
  wires:
  In1/1 -> Multiport Switch3/1
  Constant5/1 -> Multiport Switch3/8
  FAKTOR/1 -> Product/2
  Constant/1 -> Divide/2
  Divide/1 -> Out1/1
  Multiport Switch3/1 -> Product/1
  Product/1 -> Divide/1
  Constant26/1 -> Multiport Switch3/7
  Constant25/1 -> Multiport Switch3/6
  Constant20/1 -> Multiport Switch3/5
  Constant19/1 -> Multiport Switch3/4
  Constant21/1 -> Multiport Switch3/3
  Constant22/1 -> Multiport Switch3/2

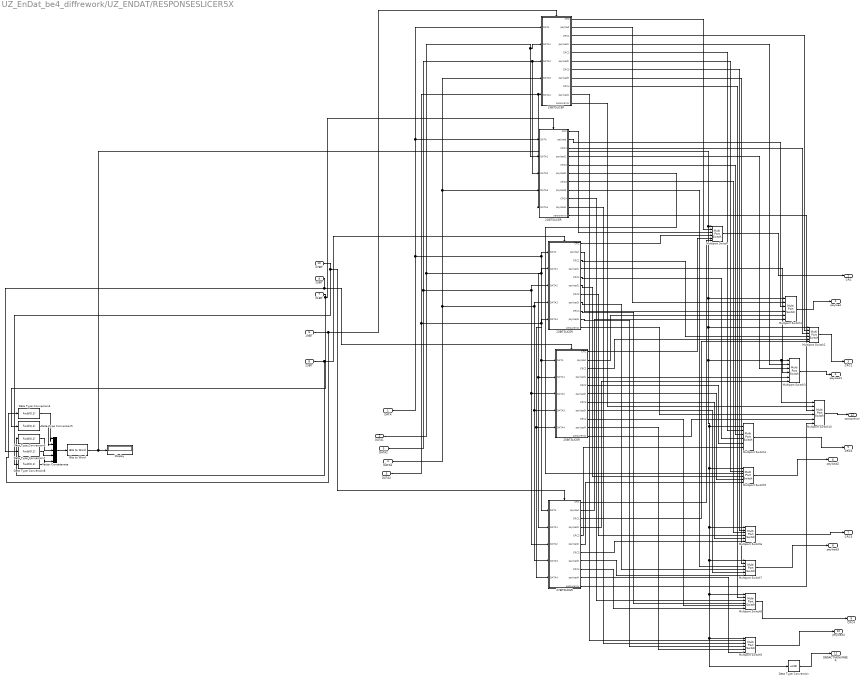
== system UZ_EnDat_be4_diffrework/UZ_ENDAT/RESPONSESLICER5X ==
  DATA : Inport
  DATA1 : Inport  Port=2
  DATA2 : Inport  Port=3
  DATA3 : Inport  Port=4
  DATA4 : Inport  Port=5
  19BIT : Inport  Port=6  OutDataTypeStr=boolean
  21BIT : Inport  Port=7  OutDataTypeStr=boolean
  23BIT : Inport  Port=8  OutDataTypeStr=boolean
  25BIT : Inport  Port=9  OutDataTypeStr=boolean
  27BIT : Inport  Port=10  OutDataTypeStr=boolean
  19BITSLICER : Subsystem
  21BITSLICER : Subsystem
  23BITSLICER : Subsystem
  25BITSLICER : Subsystem
  27BITSLICER : Subsystem
  Bits to Word : hdlsllib/Logic and Bit Operations/Bits to Word
  Data Type Conversion : DataTypeConversion  OutDataTypeStr=uint8  RndMeth=Nearest  SaturateOnIntegerOverflow=off
  Data Type Conversion{4..8} (5 alike) : DataTypeConversion  OutMax=1  OutDataTypeStr=fixdt(0,1)  SaturateOnIntegerOverflow=off  RndMeth=Floor
  Display : Display
  Multiport Switch{,1..10} (11 alike) : MultiPortSwitch  DataPortOrder=Specify indices  Inputs=5  DataPortIndices={1,2,4,8,16}  DiagnosticForDefault=Warning  SaturateOnIntegerOverflow=off  InputSameDT=off
  Vector Concatenate : Concatenate  NumInputs=5
  CRC : Outport
  payload : Outport  Port=2
  CRC1 : Outport  Port=3
  payload1 : Outport  Port=4
  CRC2 : Outport  Port=5
  payload2 : Outport  Port=6
  CRC3 : Outport  Port=7
  payload3 : Outport  Port=8
  CRC4 : Outport  Port=9
  payload4 : Outport  Port=10
  DBGACTIVENUMBER : Outport  Port=11
  sensorerror : Outport  Port=12  OutDataTypeStr=boolean
  wires:
  Multiport Switch8/1 -> CRC4/1
  23BITSLICER/1(CRC) -> Multiport Switch/4
  Multiport Switch7/1 -> payload3/1
  Multiport Switch9/1 -> payload4/1
  DATA1/1 -> 19BITSLICER/2(DATA1), 21BITSLICER/2(DATA1), 23BITSLICER/2(DATA1), 27BITSLICER/2(DATA1), 25BITSLICER/2(DATA1)
  DATA4/1 -> 21BITSLICER/5(DATA4), 19BITSLICER/5(DATA4), 23BITSLICER/5(DATA4), 27BITSLICER/5(DATA4), 25BITSLICER/5(DATA4)
  DATA2/1 -> 21BITSLICER/3(DATA2), 19BITSLICER/3(DATA2), 23BITSLICER/3(DATA2), 27BITSLICER/3(DATA2), 25BITSLICER/3(DATA2)
  DATA3/1 -> 19BITSLICER/4(DATA3), 21BITSLICER/4(DATA3), 23BITSLICER/4(DATA3), 27BITSLICER/4(DATA3), 25BITSLICER/4(DATA3)
  DATA/1 -> 19BITSLICER/1(DATA), 21BITSLICER/1(DATA), 23BITSLICER/1(DATA), 27BITSLICER/1(DATA), 25BITSLICER/1(DATA)
  Multiport Switch2/1 -> CRC1/1
  Multiport Switch3/1 -> payload1/1
  Multiport Switch4/1 -> CRC2/1
  Multiport Switch5/1 -> payload2/1
  Multiport Switch1/1 -> payload/1
  Multiport Switch6/1 -> CRC3/1
  Bits to Word/1 -> Data Type Conversion/1, Multiport Switch9/1, Multiport Switch8/1, Multiport Switch7/1, Multiport Switch6/1, Multiport Switch5/1, Multiport Switch4/1, Multiport Switch10/1, Multiport Switch3/1, Multiport Switch2/1, Multiport Switch1/1, Multiport Switch/1, Display/1
  Multiport Switch/1 -> CRC/1
  19BIT/1 -> 19BITSLICER/Enable, Data Type Conversion4/1
  Data Type Conversion6/1 -> Vector Concatenate/3
  25BIT/1 -> Data Type Conversion7/1, 25BITSLICER/Enable
  Vector Concatenate/1 -> Bits to Word/1
  23BIT/1 -> 23BITSLICER/Enable, Data Type Conversion6/1
  Data Type Conversion4/1 -> Vector Concatenate/1
  Data Type Conversion7/1 -> Vector Concatenate/4
  27BIT/1 -> 27BITSLICER/Enable, Data Type Conversion8/1
  Data Type Conversion5/1 -> Vector Concatenate/2
  21BIT/1 -> 21BITSLICER/Enable, Data Type Conversion5/1
  Data Type Conversion8/1 -> Vector Concatenate/5
  19BITSLICER/1(CRC) -> Multiport Switch/2
  21BITSLICER/1(CRC) -> Multiport Switch/3
  25BITSLICER/1(CRC) -> Multiport Switch/5
  27BITSLICER/1(CRC) -> Multiport Switch/6
  23BITSLICER/2(payload) -> Multiport Switch1/4
  19BITSLICER/2(payload) -> Multiport Switch1/2
  21BITSLICER/2(payload) -> Multiport Switch1/3
  25BITSLICER/2(payload) -> Multiport Switch1/5
  27BITSLICER/2(payload) -> Multiport Switch1/6
  23BITSLICER/3(CRC1) -> Multiport Switch2/4
  21BITSLICER/3(CRC1) -> Multiport Switch2/3
  19BITSLICER/3(CRC1) -> Multiport Switch2/2
  25BITSLICER/3(CRC1) -> Multiport Switch2/5
  27BITSLICER/3(CRC1) -> Multiport Switch2/6
  23BITSLICER/4(payload1) -> Multiport Switch3/4
  21BITSLICER/4(payload1) -> Multiport Switch3/3
  19BITSLICER/4(payload1) -> Multiport Switch3/2
  25BITSLICER/4(payload1) -> Multiport Switch3/5
  27BITSLICER/4(payload1) -> Multiport Switch3/6
  23BITSLICER/5(CRC2) -> Multiport Switch4/4
  19BITSLICER/5(CRC2) -> Multiport Switch4/2
  21BITSLICER/5(CRC2) -> Multiport Switch4/3
  25BITSLICER/5(CRC2) -> Multiport Switch4/5
  27BITSLICER/5(CRC2) -> Multiport Switch4/6
  23BITSLICER/6(payload2) -> Multiport Switch5/4
  19BITSLICER/6(payload2) -> Multiport Switch5/2
  21BITSLICER/6(payload2) -> Multiport Switch5/3
  25BITSLICER/6(payload2) -> Multiport Switch5/5
  27BITSLICER/6(payload2) -> Multiport Switch5/6
  23BITSLICER/7(CRC3) -> Multiport Switch6/4
  27BITSLICER/7(CRC3) -> Multiport Switch6/6
  25BITSLICER/7(CRC3) -> Multiport Switch6/5
  19BITSLICER/7(CRC3) -> Multiport Switch6/2
  21BITSLICER/7(CRC3) -> Multiport Switch6/3
  27BITSLICER/8(payload3) -> Multiport Switch7/6
  25BITSLICER/8(payload3) -> Multiport Switch7/5
  23BITSLICER/8(payload3) -> Multiport Switch7/4
  21BITSLICER/8(payload3) -> Multiport Switch7/3
  19BITSLICER/8(payload3) -> Multiport Switch7/2
  27BITSLICER/9(CRC4) -> Multiport Switch8/6
  25BITSLICER/9(CRC4) -> Multiport Switch8/5
  23BITSLICER/9(CRC4) -> Multiport Switch8/4
  21BITSLICER/9(CRC4) -> Multiport Switch8/3
  19BITSLICER/9(CRC4) -> Multiport Switch8/2
  23BITSLICER/10(payload4) -> Multiport Switch9/4
  27BITSLICER/10(payload4) -> Multiport Switch9/6
  25BITSLICER/10(payload4) -> Multiport Switch9/5
  19BITSLICER/10(payload4) -> Multiport Switch9/2
  21BITSLICER/10(payload4) -> Multiport Switch9/3
  Data Type Conversion/1 -> DBGACTIVENUMBER/1
  Multiport Switch10/1 -> sensorerror/1
  25BITSLICER/11(sensorerror) -> Multiport Switch10/5
  27BITSLICER/11(sensorerror) -> Multiport Switch10/6
  23BITSLICER/11(sensorerror) -> Multiport Switch10/4
  21BITSLICER/11(sensorerror) -> Multiport Switch10/3
  19BITSLICER/11(sensorerror) -> Multiport Switch10/2

== system UZ_EnDat_be4_diffrework/UZ_ENDAT/SetZero32modified ==
  valin : Inport
  setzero : Inport  Port=2  OutDataTypeStr=boolean
  Trigger : TriggerPort  TriggerType=either  VariantControl=(inherit)
  Constant2 : Constant  Value=0  OutDataTypeStr=Inherit: Inherit via back propagation  SampleTime=-1
  Index Vector1 : MultiPortSwitch  DataPortOrder=Zero-based contiguous  Inputs=2  zeroidx=on  OutDataTypeStr=fixdt(0,4,0)  SaturateOnIntegerOverflow=off  InputSameDT=off
  valueout : Outport  InitialOutput=1  VectorParamsAs1DForOutWhenUnconnected=off
  wires:
  valin/1 -> Index Vector1/2
  Index Vector1/1 -> valueout/1
  Constant2/1 -> Index Vector1/3
  setzero/1 -> Index Vector1/1

== system UZ_EnDat_be4_diffrework/UZ_ENDAT/SetZeroBool ==
  valin : Inport
  setzero : Inport  Port=2  OutDataTypeStr=boolean
  Trigger : TriggerPort  TriggerType=either  VariantControl=(inherit)
  Constant1 : Constant  OutDataTypeStr=boolean  SampleTime=-1
  Constant2 : Constant  Value=0  OutDataTypeStr=boolean  SampleTime=-1
  Index Vector1 : MultiPortSwitch  DataPortOrder=Zero-based contiguous  Inputs=2  zeroidx=on  SaturateOnIntegerOverflow=off  InputSameDT=off
  Logical Operator : Logic  AllPortsSameDT=off  OutDataTypeStr=boolean
  valueout : Outport  InitialOutput=1  VectorParamsAs1DForOutWhenUnconnected=off
  wires:
  Index Vector1/1 -> Logical Operator/1
  valin/1 -> Logical Operator/2
  Logical Operator/1 -> valueout/1
  Constant1/1 -> Index Vector1/2
  Constant2/1 -> Index Vector1/3
  setzero/1 -> Index Vector1/1

== system UZ_EnDat_be4_diffrework/UZ_ENDAT/SetZeroBool1 ==
  valin : Inport
  setzero : Inport  Port=2  OutDataTypeStr=boolean
  Trigger : TriggerPort  TriggerType=either  VariantControl=(inherit)
  Constant1 : Constant  OutDataTypeStr=boolean  SampleTime=-1
  Constant2 : Constant  Value=0  OutDataTypeStr=boolean  SampleTime=-1
  Index Vector1 : MultiPortSwitch  DataPortOrder=Zero-based contiguous  Inputs=2  zeroidx=on  SaturateOnIntegerOverflow=off  InputSameDT=off
  Logical Operator : Logic  AllPortsSameDT=off  OutDataTypeStr=boolean
  valueout : Outport  InitialOutput=1  VectorParamsAs1DForOutWhenUnconnected=off
  wires:
  Index Vector1/1 -> Logical Operator/1
  valin/1 -> Logical Operator/2
  Logical Operator/1 -> valueout/1
  Constant1/1 -> Index Vector1/2
  Constant2/1 -> Index Vector1/3
  setzero/1 -> Index Vector1/1

== system UZ_EnDat_be4_diffrework/UZ_ENDAT/SetZeroBool2 ==
  valin : Inport
  setzero : Inport  Port=2  OutDataTypeStr=boolean
  Trigger : TriggerPort  TriggerType=either  VariantControl=(inherit)
  Constant1 : Constant  OutDataTypeStr=boolean  SampleTime=-1
  Constant2 : Constant  Value=0  OutDataTypeStr=boolean  SampleTime=-1
  Index Vector1 : MultiPortSwitch  DataPortOrder=Zero-based contiguous  Inputs=2  zeroidx=on  SaturateOnIntegerOverflow=off  InputSameDT=off
  Logical Operator : Logic  AllPortsSameDT=off  OutDataTypeStr=boolean
  valueout : Outport  InitialOutput=1  VectorParamsAs1DForOutWhenUnconnected=off
  wires:
  Index Vector1/1 -> Logical Operator/1
  valin/1 -> Logical Operator/2
  Logical Operator/1 -> valueout/1
  Constant1/1 -> Index Vector1/2
  Constant2/1 -> Index Vector1/3
  setzero/1 -> Index Vector1/1

== system UZ_EnDat_be4_diffrework/UZ_ENDAT/SetZeroBool3 ==
  valin : Inport
  setzero : Inport  Port=2  OutDataTypeStr=boolean
  Trigger : TriggerPort  TriggerType=either  VariantControl=(inherit)
  Constant1 : Constant  OutDataTypeStr=boolean  SampleTime=-1
  Constant2 : Constant  Value=0  OutDataTypeStr=boolean  SampleTime=-1
  Index Vector1 : MultiPortSwitch  DataPortOrder=Zero-based contiguous  Inputs=2  zeroidx=on  SaturateOnIntegerOverflow=off  InputSameDT=off
  Logical Operator : Logic  AllPortsSameDT=off  OutDataTypeStr=boolean
  valueout : Outport  InitialOutput=1  VectorParamsAs1DForOutWhenUnconnected=off
  wires:
  Index Vector1/1 -> Logical Operator/1
  valin/1 -> Logical Operator/2
  Logical Operator/1 -> valueout/1
  Constant1/1 -> Index Vector1/2
  Constant2/1 -> Index Vector1/3
  setzero/1 -> Index Vector1/1

== system UZ_EnDat_be4_diffrework/UZ_ENDAT/SetZeroBool4 ==
  valin : Inport
  setzero : Inport  Port=2  OutDataTypeStr=boolean
  Trigger : TriggerPort  TriggerType=either  VariantControl=(inherit)
  Constant1 : Constant  OutDataTypeStr=boolean  SampleTime=-1
  Constant2 : Constant  Value=0  OutDataTypeStr=boolean  SampleTime=-1
  Index Vector1 : MultiPortSwitch  DataPortOrder=Zero-based contiguous  Inputs=2  zeroidx=on  SaturateOnIntegerOverflow=off  InputSameDT=off
  Logical Operator : Logic  AllPortsSameDT=off  OutDataTypeStr=boolean
  valueout : Outport  InitialOutput=1  VectorParamsAs1DForOutWhenUnconnected=off
  wires:
  Index Vector1/1 -> Logical Operator/1
  valin/1 -> Logical Operator/2
  Logical Operator/1 -> valueout/1
  Constant1/1 -> Index Vector1/2
  Constant2/1 -> Index Vector1/3
  setzero/1 -> Index Vector1/1

== system UZ_EnDat_be4_diffrework/UZ_ENDAT/SetZeroBool5 ==
  valin : Inport
  setzero : Inport  Port=2  OutDataTypeStr=boolean
  Trigger : TriggerPort  TriggerType=either  VariantControl=(inherit)
  Constant1 : Constant  OutDataTypeStr=boolean  SampleTime=-1
  Constant2 : Constant  Value=0  OutDataTypeStr=boolean  SampleTime=-1
  Index Vector1 : MultiPortSwitch  DataPortOrder=Zero-based contiguous  Inputs=2  zeroidx=on  SaturateOnIntegerOverflow=off  InputSameDT=off
  Logical Operator : Logic  AllPortsSameDT=off  OutDataTypeStr=boolean
  valueout : Outport  InitialOutput=1  VectorParamsAs1DForOutWhenUnconnected=off
  wires:
  Index Vector1/1 -> Logical Operator/1
  valin/1 -> Logical Operator/2
  Logical Operator/1 -> valueout/1
  Constant1/1 -> Index Vector1/2
  Constant2/1 -> Index Vector1/3
  setzero/1 -> Index Vector1/1

== system UZ_EnDat_be4_diffrework/UZ_ENDAT/Storage16 ==
  Data : Inport
  Write : Inport  Port=2  OutDataTypeStr=boolean
  Compare To Zero : hdlsllib/Logic and Bit Operations/Compare To Zero  relop===  OutDataTypeStr=boolean
  Logical Operator : Logic  Operator=NOT  AllPortsSameDT=off  OutDataTypeStr=boolean
  Logical Operator1 : Logic  Inputs=3  AllPortsSameDT=off  OutDataTypeStr=boolean
  Logical Operator2 : Logic  Operator=NOT  AllPortsSameDT=off  OutDataTypeStr=boolean
  Logical Operator3 : Logic  AllPortsSameDT=off  OutDataTypeStr=boolean
  Relational Operator : RelationalOperator  Operator===  OutDataTypeStr=boolean  InputSameDT=off
  Single Port RAM System : hdlsllib/HDL RAMs/Single Port RAM System  RAMType=Single port  AsyncRead=off  WriteOutputValue=Old data  RAMInitialValue=0  allowBusInputs=off  WritesHaveOutput=on  NumReads=0  NumWrites=1  SimulateUsing=Code generation
  adress : Constant  Value=5  OutDataTypeStr=uint8  SampleTime=-1
  out : Outport
  wrok : Outport  Port=2  OutDataTypeStr=boolean
  wires:
  Single Port RAM System/1 -> Relational Operator/1, out/1
  Data/1 -> Compare To Zero/1, Single Port RAM System/1, Relational Operator/2
  adress/1 -> Single Port RAM System/2
  Relational Operator/1 -> Logical Operator3/1, Logical Operator/1
  Logical Operator/1 -> Logical Operator1/2
  Write/1 -> Logical Operator1/1
  Compare To Zero/1 -> Logical Operator2/1
  Logical Operator2/1 -> Logical Operator3/2, Logical Operator1/3
  Logical Operator1/1 -> Single Port RAM System/3
  Logical Operator3/1 -> wrok/1

== system UZ_EnDat_be4_diffrework/UZ_ENDAT/Subsystem ==
  CLK : Inport
  RESET : Inport  Port=2
  CLKS2DATAFLOWCHG : Inport  Port=3
  CLK2ENDOFTRANSMISSION : Inport  Port=4
  VERYSLOWCLK : Inport  Port=5
  Constant : Constant  OutDataTypeStr=boolean  SampleTime=-1
  Constant1 : Constant  Value=0  OutDataTypeStr=boolean  SampleTime=-1
  stalebootupfunction : Subsystem  Commented=on
      settings: LibrarySourceBlock=|
      | hdlsllib/Ports &
      | Subsystems/Subsystem
  CLKOUT : Outport
  DATAOUT : Outport  Port=2
  BOOTUPCOMPLETE : Outport  Port=3
  DATAINV : Outport  Port=4
  wires:
  stalebootupfunction/1(CLKOUT) -> ?
  stalebootupfunction/3(BOOTUPCOMPLETE) -> ?
  CLK2ENDOFTRANSMISSION/1 -> stalebootupfunction/4(CLK2ENDOFTRANSMISSION)
  stalebootupfunction/4(DATAINV) -> ?
  stalebootupfunction/2(DATAOUT) -> ?
  CLK/1 -> stalebootupfunction/1(CLK)
  CLKS2DATAFLOWCHG/1 -> stalebootupfunction/3(CLKS2DATAFLOWCHG)
  VERYSLOWCLK/1 -> stalebootupfunction/5(VERYSLOWCLK)
  RESET/1 -> stalebootupfunction/2(RESET)
  Constant/1 -> DATAINV/1, BOOTUPCOMPLETE/1, CLKOUT/1
  Constant1/1 -> DATAOUT/1

== system UZ_EnDat_be4_diffrework/UZ_ENDAT/Subsystem1 ==
  in : Inport
  Enable : EnablePort
  Bits to Word1 : hdlsllib/Logic and Bit Operations/Bits to Word
  out : Outport  InitialOutput=0
  wires:
  Bits to Word1/1 -> out/1
  in/1 -> Bits to Word1/1

== system UZ_EnDat_be4_diffrework/UZ_ENDAT/Subsystem2 ==
  CLK : Inport
  SLOWCLCK : Inport  Port=2
  DATA : Inport  Port=3
  reset : Inport  Port=4
  Enable : EnablePort
  ManualDeserializere : Subsystem
      settings: LibrarySourceBlock=|
      | hdlsllib/Ports &
      | Subsystems/Subsystem
  valin : Outport  InitialOutput=0
  wires:
  CLK/1 -> ManualDeserializere/1(CLK)
  DATA/1 -> ManualDeserializere/3(DATA)
  reset/1 -> ManualDeserializere/4(reset)
  SLOWCLCK/1 -> ManualDeserializere/2(SLOWCLCK)
  ManualDeserializere/1(valin) -> valin/1

== system UZ_EnDat_be4_diffrework/UZ_ENDAT/Subsystem6 ==
  In1 : Inport  OutDataTypeStr=uint16
  FACTOR : Inport  Port=2  OutMin=0  OutMax=60000
  Constant : Constant  Value=100  OutDataTypeStr=uint16  SampleTime=-1
  Divide : Product  Inputs=*/  InputSameDT=on  OutDataTypeStr=uint16  RndMeth=Simplest  SaturateOnIntegerOverflow=on
  Product : Product  RndMeth=Simplest  SaturateOnIntegerOverflow=on  OutDataTypeStr=Inherit: Same as first input
  Out1 : Outport
  wires:
  In1/1 -> Product/1
  FACTOR/1 -> Product/2
  Constant/1 -> Divide/2
  Product/1 -> Divide/1
  Divide/1 -> Out1/1

== system UZ_EnDat_be4_diffrework/UZ_ENDAT/ramselektor ==
  In1 : Inport  OutMin=0  OutMax=15  OutDataTypeStr=fixdt(0,4,0, 'DataTypeOverride', 'Off')  LockScale=on
  Trigger : TriggerPort  VariantControl=(inherit)  OutputDataType=int8  InitialTriggerSignalState=positive
  Delay : Delay  DelayLength=99
  Increment Stored Integer : hdlsllib/Math Operations/Increment Stored Integer
  SEL : Outport  InitialOutput=0
  wires:
  In1/1 -> Delay/1
  Increment Stored Integer/1 -> SEL/1
  Delay/1 -> Increment Stored Integer/1

== system UZ_EnDat_be4_diffrework/UZ_ENDAT/responseslicer5 ==
  DATA : Inport  OutDataTypeStr=uint64
  Bit Slice : hdlsllib/Logic and Bit Operations/Bit Slice  Commented=on  lidx=15  ridx=0
  Bit Slice1 : hdlsllib/Logic and Bit Operations/Bit Slice  Commented=on  lidx=63  ridx=48
  Bit Slice2 : hdlsllib/Logic and Bit Operations/Bit Slice  Commented=on  lidx=47  ridx=44
  Bit Slice3 : hdlsllib/Logic and Bit Operations/Bit Slice  lidx=43  ridx=39
  Bit Slice4 : hdlsllib/Logic and Bit Operations/Bit Slice  lidx=38  ridx=16
  Data Type Conversion : DataTypeConversion  Commented=on  OutDataTypeStr=uint16  SaturateOnIntegerOverflow=off  RndMeth=Floor
  Data Type Conversion1 : DataTypeConversion  Commented=on  OutDataTypeStr=uint16  SaturateOnIntegerOverflow=off  RndMeth=Floor
  Data Type Conversion2 : DataTypeConversion  Commented=through  OutDataTypeStr=uint8  SaturateOnIntegerOverflow=off  RndMeth=Floor
  Data Type Conversion3 : DataTypeConversion  OutDataTypeStr=uint8  SaturateOnIntegerOverflow=off  RndMeth=Floor
  Data Type Conversion4 : DataTypeConversion  OutDataTypeStr=uint32  SaturateOnIntegerOverflow=off  RndMeth=Floor
  ENDAT23BITREVERSER : Subsystem  Commented=on
  upppadding : Outport  OutDataTypeStr=uint16
  lowpadding : Outport  Port=2  OutDataTypeStr=uint16
  upperrecivervalue : Outport  Port=3  OutDataTypeStr=uint8
  CRC : Outport  Port=4  OutDataTypeStr=uint8
  payload : Outport  Port=5  OutDataTypeStr=uint32
  wires:
  DATA/1 -> Bit Slice4/1, Bit Slice3/1
  Bit Slice/1 -> Data Type Conversion/1
  Bit Slice1/1 -> Data Type Conversion1/1
  Data Type Conversion/1 -> lowpadding/1
  Data Type Conversion1/1 -> upppadding/1
  Bit Slice3/1 -> Data Type Conversion3/1
  Bit Slice2/1 -> Data Type Conversion2/1
  Bit Slice4/1 -> ENDAT23BITREVERSER/1(in), Data Type Conversion4/1
  Data Type Conversion2/1 -> upperrecivervalue/1
  Data Type Conversion3/1 -> CRC/1
  Data Type Conversion4/1 -> payload/1

== system UZ_EnDat_be4_diffrework/UZ_ENDAT/timingprovider ==
  wrok : Inport  OutDataTypeStr=boolean
  clk : Inport  Port=2  OutDataTypeStr=boolean
  CLKCNTER_POSCNTR : Subsystem
      settings: LibrarySourceBlock=|
      | hdlsllib/Ports &
      | Subsystems/Subsystem
  CLKCNTER_POSCNTR1 : Subsystem
      settings: LibrarySourceBlock=|
      | hdlsllib/Ports &
      | Subsystems/Subsystem
  Compare To Constant : hdlsllib/Logic and Bit Operations/Compare To Constant  relop=>  const=5  OutDataTypeStr=boolean
  Compare To Constant1 : hdlsllib/Logic and Bit Operations/Compare To Constant  relop===  const=0  OutDataTypeStr=boolean
  Constant3 : Constant  Commented=on  Value=0x7FFFF0  OutDataTypeStr=uint32  SampleTime=-1
  Constant4 : Constant  Commented=on  Value=0x7FFFFF  OutDataTypeStr=uint32  SampleTime=-1
  Detect Increase1 : simulink/Logic and Bit Operations/Detect Increase  vinit=0.0  OutDataTypeStr=boolean
      settings: LibrarySourceBlock=|
      | hdlsllib/Logic and Bit
      | Operations/Detect
      | Increase
  Logical Operator : Logic  Operator=OR  AllPortsSameDT=off  OutDataTypeStr=boolean
  Scope : Scope  NumInputPorts=2
  Subsystem : Subsystem
  Subsystem1 : Subsystem
  Subsystem2 : Subsystem
  Subsystem3 : Subsystem
  Subsystem4 : Subsystem  Commented=on
  timeelapsed4cycl : Outport  OutDataTypeStr=uint32
  timeelapsed3cycl : Outport  Port=2  OutDataTypeStr=uint32
  timeelapsed2cycl : Outport  Port=3  OutDataTypeStr=uint32
  timeelapsed1cycl : Outport  Port=4  OutDataTypeStr=uint32
  wires:
  clk/1 -> CLKCNTER_POSCNTR1/1(CLK), Subsystem4/1(countclk), CLKCNTER_POSCNTR/2(CLK2CNT), CLKCNTER_POSCNTR/1(CLK)
  wrok/1 -> Detect Increase1/1
  Detect Increase1/1 -> CLKCNTER_POSCNTR1/2(CLK2CNT)
  Subsystem/1(ns elapsed) -> timeelapsed4cycl/1
  CLKCNTER_POSCNTR/1(CNT) -> Subsystem3/2(clkcnt), Subsystem2/2(clkcnt), Subsystem1/2(clkcnt), Scope/2, Subsystem/2(clkcnt)
  Subsystem1/1(ns elapsed) -> timeelapsed3cycl/1
  Subsystem2/1(ns elapsed) -> timeelapsed2cycl/1
  Subsystem3/1(ns elapsed) -> timeelapsed1cycl/1
  CLKCNTER_POSCNTR1/1(CNT) -> Scope/1, Subsystem3/1(elapsed), Subsystem2/1(elapsed), Subsystem1/1(elapsed), Subsystem/1(elapsed), Compare To Constant/1, Compare To Constant1/1
  Compare To Constant/1 -> Logical Operator/1, CLKCNTER_POSCNTR1/3(ResetCNT)
  Logical Operator/1 -> Subsystem4/2(reset), CLKCNTER_POSCNTR/3(ResetCNT)
  Compare To Constant1/1 -> Logical Operator/2

== system UZ_EnDat_be4_diffrework/UZ_ENDAT/5timestorage/Storage1 ==
  Data : Inport
  Write : Inport  Port=2  OutDataTypeStr=boolean
  Delay2 : Delay  DelayLength=1
  Switch : Switch  Criteria=u2 > Threshold  SaturateOnIntegerOverflow=off  InputSameDT=off
  out : Outport
  wires:
  Switch/1 -> Delay2/1, out/1
  Delay2/1 -> Switch/3
  Data/1 -> Switch/1
  Write/1 -> Switch/2

== system UZ_EnDat_be4_diffrework/UZ_ENDAT/5timestorage/Storage2 ==
  Data : Inport
  Write : Inport  Port=2  OutDataTypeStr=boolean
  Delay2 : Delay  DelayLength=1
  Switch : Switch  Criteria=u2 > Threshold  SaturateOnIntegerOverflow=off  InputSameDT=off
  out : Outport
  wires:
  Switch/1 -> Delay2/1, out/1
  Delay2/1 -> Switch/3
  Data/1 -> Switch/1
  Write/1 -> Switch/2

== system UZ_EnDat_be4_diffrework/UZ_ENDAT/5timestorage/Storage20 ==
  Data : Inport
  Write : Inport  Port=2  OutDataTypeStr=boolean
  Delay2 : Delay  DelayLength=1
  Switch : Switch  Criteria=u2 > Threshold  SaturateOnIntegerOverflow=off  InputSameDT=off
  out : Outport
  wires:
  Switch/1 -> Delay2/1, out/1
  Delay2/1 -> Switch/3
  Data/1 -> Switch/1
  Write/1 -> Switch/2

== system UZ_EnDat_be4_diffrework/UZ_ENDAT/5timestorage/Storage3 ==
  Data : Inport
  Write : Inport  Port=2  OutDataTypeStr=boolean
  Delay2 : Delay  DelayLength=1
  Switch : Switch  Criteria=u2 > Threshold  SaturateOnIntegerOverflow=off  InputSameDT=off
  out : Outport
  wires:
  Switch/1 -> Delay2/1, out/1
  Delay2/1 -> Switch/3
  Data/1 -> Switch/1
  Write/1 -> Switch/2
